simulink model "Kalman_Simulink"  (R2019b)
settings: Solver=VariableStepAuto  StartTime=0.0  StopTime=3  FixedStep=0.01  RelTol=1e-3
values from neighbouring files (symbols this model uses):
  A = [Ae zeros(p, ro); zeros(ro, p) At]    [Kalman.m]    (also in Kalman_EMG.m)
  B = [zeros(p, 1); Bt]    [Kalman.m]    (also in Kalman_EMG.m)
  C = [Ce Ct]    [Kalman.m]    (also in Kalman_EMG.m)
  Q = [sigmaE zeros(1, ro); zeros(ro, 1) sigmaT2*eye(ro)]    [Kalman.m]    (also in Kalman_EMG.m = zeros(30000*(ro+1), ro+1))
  R = sigmaV    [Kalman.m]    (also in Kalman_EMG.m = zeros(1, 30000))
  Ts = y_arm.interval    [Kalman.m]    (also in Kalman_EMG.m)
undefined symbols (not defined in the file or in its folder): Discrete, Time
libraries: dspsrcs4 x4, ctrlSharedLib x1
settings Model: Creator=mulusoy  LastModifiedBy=isidoraradenkovic
settings DataIOCC: ReturnWorkspaceOutputs=off
settings OptimizationCC: DefaultParameterBehavior=Inlined  PassReuseOutputArgsAs=Individual arguments  EfficientTunableParamExpr=on
settings DebuggingCC: ParameterTunabilityLossMsg=error  ArithmeticOperatorsInVariantConditions=warning
settings SFSimCC: SimUseLocalCustomCode=off  MATLABDynamicMemAlloc=off  CustomCodeUndefinedFunction=UseInterfaceOnly
settings RTWCC: SystemTargetFile=ert.tlc  TemplateMakefile=ert_default_tmf  GenerateReport=on  RTWUseLocalCustomCode=off  IncludeHyperlinkInReport=on  LaunchReport=on  GenerateTraceInfo=on  GenerateTraceReport=on  GenerateTraceReportSl=on  GenerateTraceReportSf=on  GenerateTraceReportEml=on  CheckMdlBeforeBuild=Warning
settings CodeAppCC: GenerateComments=off  IgnoreCustomStorageClasses=off  SimulinkBlockComments=off
settings ERTTargetCC: TargetLangStandard=C99 (ISO)  GenerateSampleERTMain=on  InlinedParameterPlacement=NonHierarchical  ERTCustomFileTemplate=example_file_process.tlc
settings SimscapeCC: SimscapeNormalizeSystem=off

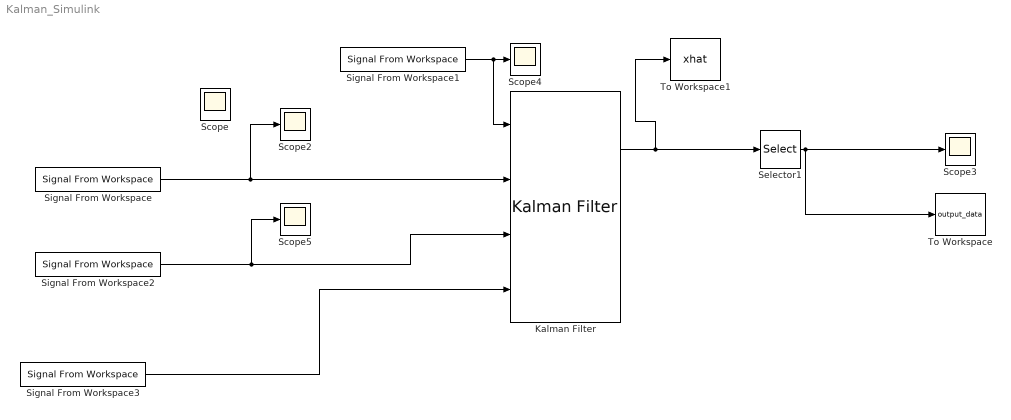
== system Kalman_Simulink ==
  Kalman Filter : ctrlSharedLib/Kalman Filter  TimeDomain=Discrete-Time  UseCurrentEstimator=on  ModelSource=Individual A, B, C, D matrices  ModelSourceVariable=ss(0.95,1,1,0,1)  A=A  B=B  C=C  D=0  NumberOfStates=1  NumberOfInputs=1  NumberOfOutputs=1  InitialEstimateSource=Dialog  X0=[0.3 0 0 0 0 0]  P0=1  UseK=off  UseGH=on  NumberOfProcessNoiseInputs=1  G=G  TimeInvariantG=on  H=0  TimeInvariantH=on  Q=diag([0,Q])  TimeInvariantQ=off  R=R  TimeInvariantR=off  N=0  TimeInvariantN=on  AddInputPort=on  AddEnablePort=off  OutputEstimatedY=off  OutputP=on  Ts=Ts
      settings: SourceProductBaseCode=CT
  Scope{,2..5} (5 alike) : Scope
  Selector1 : Selector  InputPortWidth=6  IndexOptions=Index vector (dialog)  Indices=[1]  OutputSizes=1
  Signal From Workspace : dspsrcs4/Signal From Workspace  X=input_data  Ts=Ts  nsamps=1  OutputAfterFinalValue=Cyclic repetition  ignoreOrWarnInputAndFrameLengths=off  OutputFrames=off
  Signal From Workspace1 : dspsrcs4/Signal From Workspace  X=tms_pulses  Ts=Ts  nsamps=1  OutputAfterFinalValue=Cyclic repetition  ignoreOrWarnInputAndFrameLengths=off  OutputFrames=off
  Signal From Workspace2 : dspsrcs4/Signal From Workspace  X=Q  Ts=Ts/4  nsamps=4  OutputAfterFinalValue=Cyclic repetition  ignoreOrWarnInputAndFrameLengths=off  OutputFrames=off
  Signal From Workspace3 : dspsrcs4/Signal From Workspace  X=R  Ts=Ts  nsamps=1  OutputAfterFinalValue=Cyclic repetition  ignoreOrWarnInputAndFrameLengths=off  OutputFrames=off
  To Workspace : ToWorkspace  VariableName=output_data  SampleTime=-1
      settings: Save2DSignal=2-D array (concatenate along first dimension)
  To Workspace1 : ToWorkspace  VariableName=xhat  SampleTime=-1
      settings: Save2DSignal=2-D array (concatenate along first dimension)
  wires:
  Signal From Workspace/1 -> Kalman Filter/2, Scope2/1
  Selector1/1 -> To Workspace/1, Scope3/1
  Signal From Workspace2/1 -> Kalman Filter/3, Scope5/1
  Signal From Workspace3/1 -> Kalman Filter/4
  Signal From Workspace1/1 -> Scope4/1, Kalman Filter/1
  Kalman Filter/1 -> To Workspace1/1, Selector1/1
